simulink model "CicloCompraFase_2"  (R2024b)
settings: Solver=VariableStepAuto  StartTime=0.0  StopTime=Inf  RelTol=1e-3

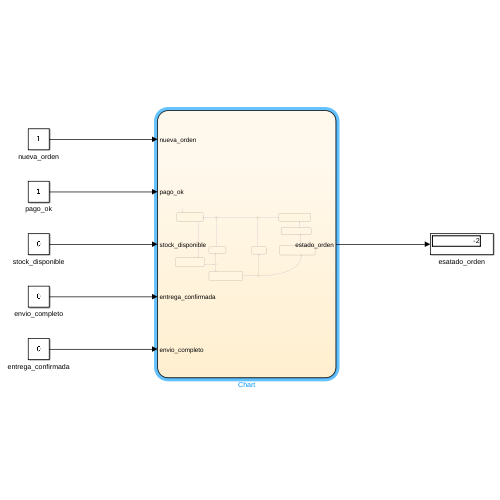
[thumbnail: Simulink's stored preview of the top-level diagram]
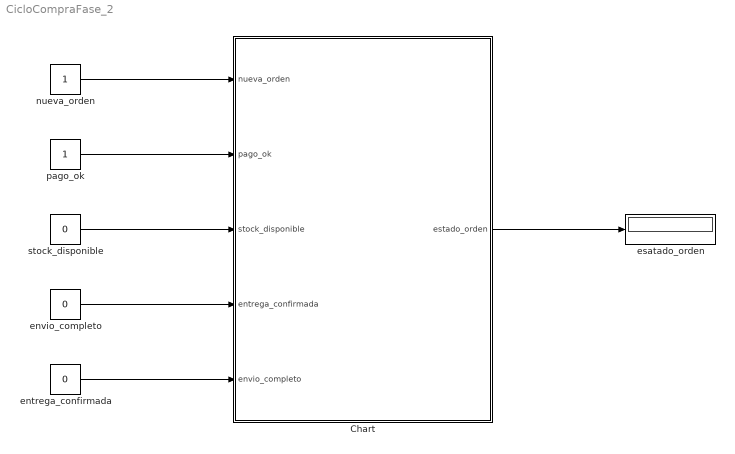
== system CicloCompraFase_2 ==
  Chart : Stateflow chart  TreatAsAtomicUnit=on
  entrega_confirmada : Constant  Value=0
  envio_completo : Constant  Value=0
  esatado_orden : Display
  nueva_orden : Constant
  pago_ok : Constant
  stock_disponible : Constant  Value=0
  wires:
  Chart/1(estado_orden) -> esatado_orden/1
  nueva_orden/1 -> Chart/1(nueva_orden)
  pago_ok/1 -> Chart/2(pago_ok)
  stock_disponible/1 -> Chart/3(stock_disponible)
  envio_completo/1 -> Chart/4(entrega_confirmada)
  entrega_confirmada/1 -> Chart/5(envio_completo)

== stateflow chart CicloCompraFase_2/Chart ==
  state Inactivo
    entry:
    estado_orden=0
  state Orden_Entregada
    entry:
    estado_orden=5
  state Orden_Enviada
    entry:
    estado_orden=4
  state Inventario_Asignado
    entry:
    estado_orden=3
  state Pago_Fallido
    entry:
    estado_orden=-1;
  state Fuera_de_Stock
    entry:
    estado_orden=-2;
  state Recibida
    entry:
    estado_orden=1
  state Pago_Verificado
    entry:
    estado_orden=2
  (default) -> Inactivo
  (junction 34) -> Inactivo
  (junction 35) -> (junction 34)
  Orden_Entregada -> (junction 35) : [after(5,sec)]
  Pago_Fallido -> (junction 34) : [after(5,sec)]
  Fuera_de_Stock -> (junction 35) : [after(5,sec)]
  Orden_Enviada -> Orden_Entregada : [entrega_confirmada==1]
  Inactivo -> Recibida : [nueva_orden==1]
  Inventario_Asignado -> Orden_Enviada : [envio_completo==1]
  (junction 21) -> Pago_Fallido [order 2] : [pago_ok~=1]
  (junction 26) -> Fuera_de_Stock [order 1] : [stock_disponible~=1]
  (junction 26) -> Inventario_Asignado [order 2] : [stock_disponible==1]
  Recibida -> (junction 21)
  (junction 21) -> Pago_Verificado [order 1] : [pago_ok==1]
  Pago_Verificado -> (junction 26)
  data: nueva_orden input; pago_ok input; stock_disponible input; entrega_confirmada input; envio_completo input; estado_orden output
